simulink model "Simulink_Tutorial_Youtube"  (R2022b)
settings: Solver=FixedStepAuto  StartTime=0.0  StopTime=10  FixedStep=1  RelTol=1e-3
model workspace (MAT data in the model file):
  Sig = Simulink.Signal
  Sig.DataType = 'auto'
  Sig.Dimensions = -1
  Sig.DimensionsMode = 'auto'
  Sig.Complexity = 'auto'
  Sig.SampleTime = -1
  Sig.SamplingMode = 'auto'
  pi = Simulink.Parameter
  pi.Value = 3.14
  pi.DataType = 'double'
  pi.Complexity = 'real'
  pi.Dimensions = [1 1]
undefined symbols (not defined in the file or in its folder): sigbuilder_block, valueOfCounter
libraries: simulink x15, simulink_extras x1, lib_sample x1, dspsigops x1, SignalEditorBlockLib x1
settings Model: Creator=mohsa  LastModifiedBy=mohsa

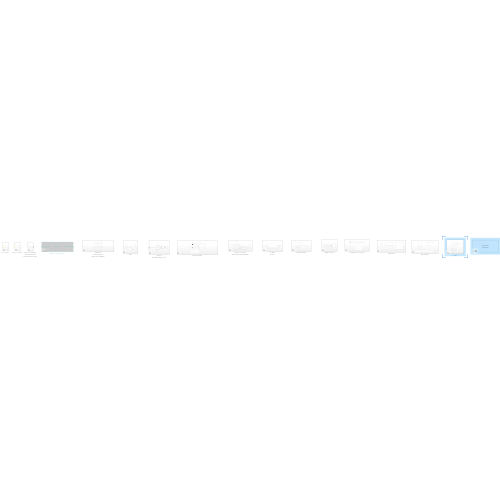
[thumbnail: Simulink's stored preview of the top-level diagram]
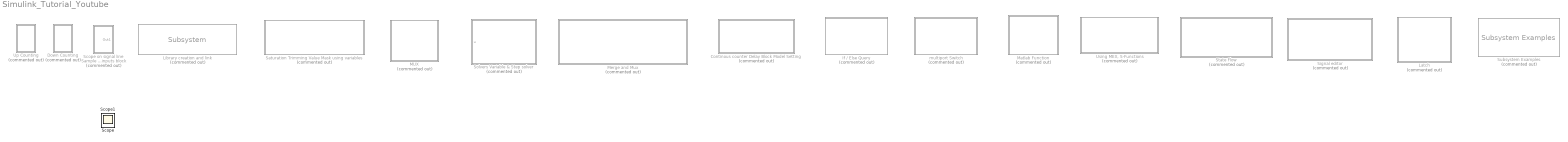
== system Simulink_Tutorial_Youtube ==
  Continous counter Delay Block Model Setting : Subsystem  Commented=on
  Down Counting : Subsystem  Commented=on
  "If / Else Query " : Subsystem  Commented=on
  Latch : Subsystem  Commented=on
  Library creation and link : lib_sample/Subsystem  Commented=on
      settings: LibrarySourceBlock=lib_sample2/Subsystem
  MUX : Subsystem  Commented=on
  Matlab Function : Subsystem  Commented=on
  Merge and Mux : Subsystem  Commented=on
  Saturation Trimming Value Mask using variables : Subsystem  Commented=on
  Scope on signal line Sample and hold Discreate inputs block : Subsystem  Commented=on
  Signal editor : Subsystem  Commented=on
  "Solvers Variable & Step solver " : Subsystem  Commented=on
  State Flow : Subsystem  Commented=on
  Subsystem Examples : simulink/Ports & Subsystems/Subsystem Examples  Commented=on
  Up Counting : Subsystem  Commented=on
  "Using MEX, S-Functions " : Subsystem  Commented=on
  multiport Switch : Subsystem  Commented=on
  Scope : Scope
  Scope1 : Scope

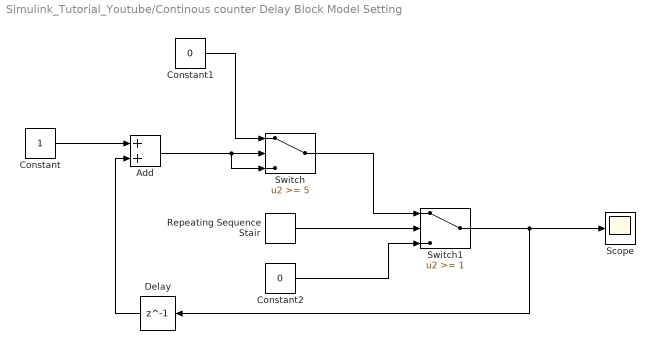
== system Simulink_Tutorial_Youtube/Continous counter Delay Block Model Setting ==
  Add : Sum
  Constant : Constant
  Constant1 : Constant  Value=0
  Constant2 : Constant  Value=0
  Delay : Delay  DelayLength=1
  Repeating Sequence Stair : simulink/Sources/Repeating Sequence Stair  OutValues=[1 ].'  tsamp=-1  OutMin=[]  OutMax=[]  OutDataTypeStr=double  OutputDataTypeScalingMode=double  OutDataType=fixdt(0,8)  ConRadixGroup=Best Precision: Vector-wise  OutScaling=2^-12
  Scope : Scope
  Switch : Switch  Threshold=5  SaturateOnIntegerOverflow=off  InputSameDT=off
  Switch1 : Switch  Threshold=1  SaturateOnIntegerOverflow=off  InputSameDT=off
  wires:
  Constant2/1 -> Switch1/3
  Repeating Sequence Stair/1 -> Switch1/2
  Switch/1 -> Switch1/1
  Constant1/1 -> Switch/1
  Add/1 -> Switch/3, Switch/2
  Constant/1 -> Add/1
  Switch1/1 -> Delay/1, Scope/1
  Delay/1 -> Add/2

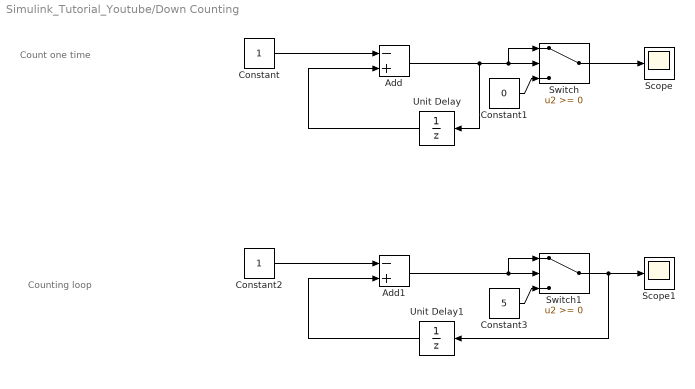
== system Simulink_Tutorial_Youtube/Down Counting ==
  note: Count one time
  note: Counting loop
  Add : Sum  Inputs=-+
  Add1 : Sum  Inputs=-+
  Constant : Constant
  Constant1 : Constant  Value=0
  Constant2 : Constant
  Constant3 : Constant  Value=5
  Scope : Scope
  Scope1 : Scope
  Switch : Switch  SaturateOnIntegerOverflow=off  InputSameDT=off
  Switch1 : Switch  SaturateOnIntegerOverflow=off  InputSameDT=off
  Unit Delay : UnitDelay  InitialCondition=valueOfCounter+1  SampleTime=-1  HasFrameUpgradeWarning=on
  Unit Delay1 : UnitDelay  InitialCondition=valueOfCounter+1  SampleTime=-1  HasFrameUpgradeWarning=on
  wires:
  Unit Delay/1 -> Add/2
  Constant/1 -> Add/1
  Switch/1 -> Scope/1
  Add/1 -> Unit Delay/1, Switch/1, Switch/2
  Constant1/1 -> Switch/3
  Constant3/1 -> Switch1/3
  Add1/1 -> Switch1/2, Switch1/1
  Switch1/1 -> Unit Delay1/1, Scope1/1
  Constant2/1 -> Add1/1
  Unit Delay1/1 -> Add1/2

== system Simulink_Tutorial_Youtube/If // Else Query  ==
  Repeating Sequence Stair : simulink/Sources/Repeating Sequence Stair  OutValues=[0:10:360].'  tsamp=-1  OutMin=[]  OutMax=[]  OutDataTypeStr=double  OutputDataTypeScalingMode=double  OutDataType=fixdt(0,8)  ConRadixGroup=Best Precision: Vector-wise  OutScaling=2^-12
  Scope : Scope  NumInputPorts=2
  Subsystem : Subsystem  mask{upperVal=3*pi/2, lowerVal=pi/2}
      mask prompts: upperVal "upper"; lowerVal "lower"
  wires:
  Repeating Sequence Stair/1 -> Scope/2, Subsystem/1(In1)
  Subsystem/1(Out1) -> Scope/1

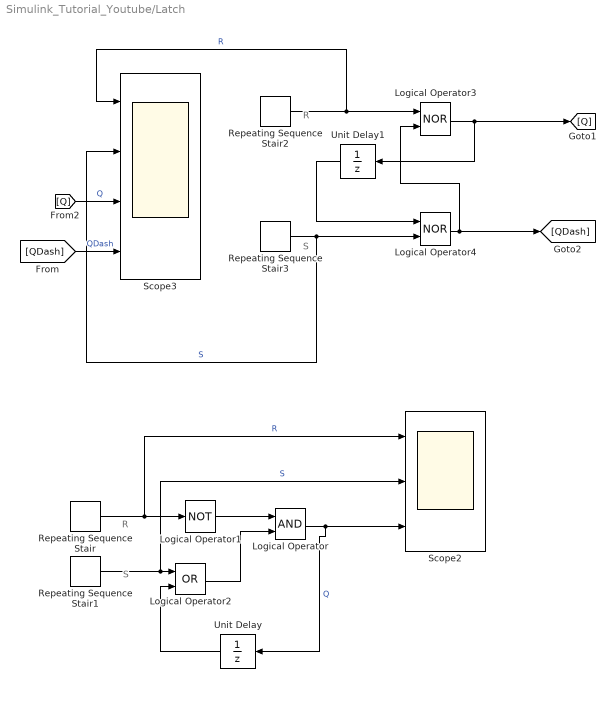
== system Simulink_Tutorial_Youtube/Latch ==
  note: S
  note: R
  note: R
  note: S
  Logical Operator : Logic  AllPortsSameDT=off  OutDataTypeStr=boolean
  Logical Operator1 : Logic  Operator=NOT  AllPortsSameDT=off  OutDataTypeStr=boolean
  Logical Operator2 : Logic  Operator=OR  AllPortsSameDT=off  OutDataTypeStr=boolean
  Logical Operator3 : Logic  Operator=NOR  AllPortsSameDT=off  OutDataTypeStr=boolean
  Logical Operator4 : Logic  Operator=NOR  AllPortsSameDT=off  OutDataTypeStr=boolean
  Repeating Sequence Stair : simulink/Sources/Repeating Sequence Stair  OutValues=[0 1 0 0 0 0 0].'  tsamp=-1  OutMin=[]  OutMax=[]  OutDataTypeStr=double  OutputDataTypeScalingMode=double  OutDataType=fixdt(0,8)  ConRadixGroup=Best Precision: Vector-wise  OutScaling=2^-12
  Repeating Sequence Stair1 : simulink/Sources/Repeating Sequence Stair  OutValues=[0 0 0 0 0 1 0].'  tsamp=-1  OutMin=[]  OutMax=[]  OutDataTypeStr=double  OutputDataTypeScalingMode=double  OutDataType=fixdt(0,8)  ConRadixGroup=Best Precision: Vector-wise  OutScaling=2^-12
  Repeating Sequence Stair2 : simulink/Sources/Repeating Sequence Stair  OutValues=[0 1 0 0 0 0 0].'  tsamp=-1  OutMin=[]  OutMax=[]  OutDataTypeStr=double  OutputDataTypeScalingMode=double  OutDataType=fixdt(0,8)  ConRadixGroup=Best Precision: Vector-wise  OutScaling=2^-12
  Repeating Sequence Stair3 : simulink/Sources/Repeating Sequence Stair  OutValues=[0 0 0 0 0 1 0].'  tsamp=-1  OutMin=[]  OutMax=[]  OutDataTypeStr=double  OutputDataTypeScalingMode=double  OutDataType=fixdt(0,8)  ConRadixGroup=Best Precision: Vector-wise  OutScaling=2^-12
  Scope2 : Scope  NumInputPorts=3
  Scope3 : Scope  NumInputPorts=4
  Unit Delay : UnitDelay  SampleTime=-1  HasFrameUpgradeWarning=on
  Unit Delay1 : UnitDelay  InitialCondition=1  SampleTime=-1  HasFrameUpgradeWarning=on
  wires:
  Logical Operator/1 -> Unit Delay/1, Scope2/3  "Q"
  Repeating Sequence Stair2/1 -> Scope3/1, Logical Operator3/1  "R"
  Repeating Sequence Stair/1 -> Scope2/1, Logical Operator1/1  "R"
  Logical Operator2/1 -> Logical Operator/2
  Unit Delay/1 -> Logical Operator2/2
  Logical Operator4/1 -> Logical Operator3/2, [QDash]
  Repeating Sequence Stair3/1 -> Scope3/2, Logical Operator4/2  "S"
  Repeating Sequence Stair1/1 -> Scope2/2, Logical Operator2/1  "S"
  Logical Operator3/1 -> Unit Delay1/1, [Q]
  [Q] -> Scope3/3  "Q"
  Logical Operator1/1 -> Logical Operator/1
  [QDash] -> Scope3/4  "QDash"
  Unit Delay1/1 -> Logical Operator4/1

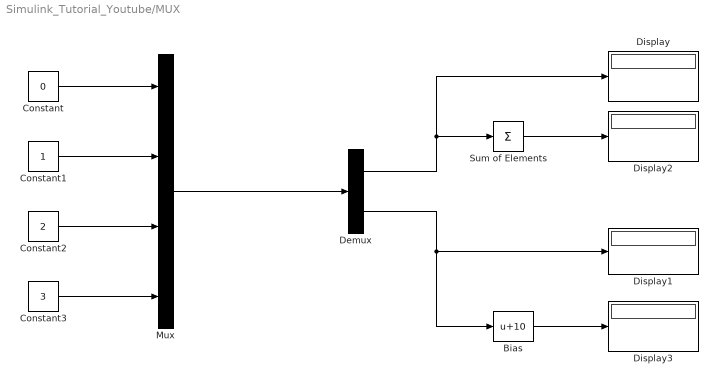
== system Simulink_Tutorial_Youtube/MUX ==
  Bias : Bias  Bias=10  SaturateOnIntegerOverflow=off
  Constant : Constant  Value=0
  Constant1 : Constant
  Constant2 : Constant  Value=2
  Constant3 : Constant  Value=3
  Demux : Demux  Outputs=2
  Display{,1..3} (4 alike) : Display
  Mux : Mux
  Sum of Elements : Sum  Inputs=+
  wires:
  Constant/1 -> Mux/1
  Constant1/1 -> Mux/2
  Constant2/1 -> Mux/3
  Constant3/1 -> Mux/4
  Mux/1 -> Demux/1
  Demux/1 -> Sum of Elements/1, Display/1
  Demux/2 -> Bias/1, Display1/1
  Sum of Elements/1 -> Display2/1
  Bias/1 -> Display3/1

== system Simulink_Tutorial_Youtube/Matlab Function ==
  MATLAB Function : MATLAB Function  TreatAsAtomicUnit=on
  Repeating Sequence Stair : simulink/Sources/Repeating Sequence Stair  OutValues=[0:10:50].'  tsamp=-1  OutMin=[]  OutMax=[]  OutDataTypeStr=double  OutputDataTypeScalingMode=double  OutDataType=fixdt(0,8)  ConRadixGroup=Best Precision: Vector-wise  OutScaling=2^-12
  Scope : Scope  NumInputPorts=4
  wires:
  Repeating Sequence Stair/1 -> Scope/1, MATLAB Function/1(u)
  MATLAB Function/1(x) -> Scope/2
  MATLAB Function/2(y) -> Scope/3
  MATLAB Function/3(z) -> Scope/4

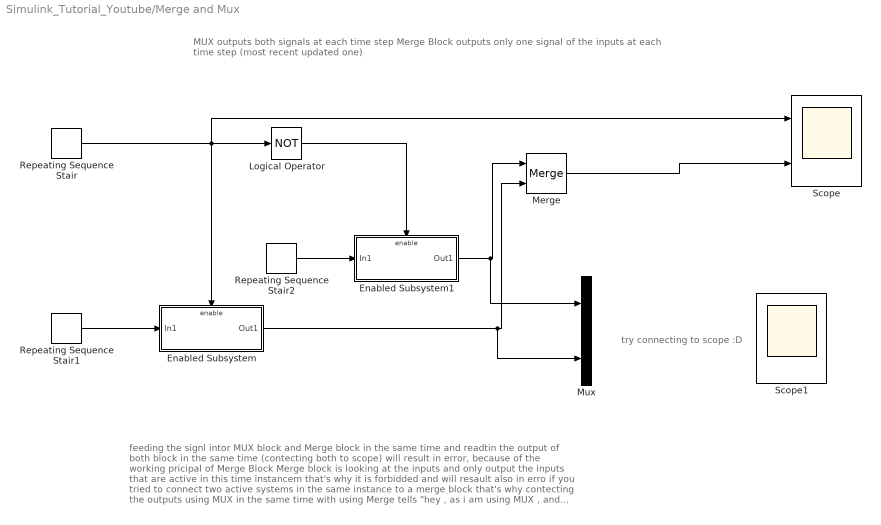
== system Simulink_Tutorial_Youtube/Merge and Mux ==
  note: MUX outputs both signals at each time step
      | Merge Block outputs only one signal of the inputs at each time step (most recent updated one)
  note: try connecting to scope :D
  note: feeding the signl intor MUX block and Merge block in the same time and readtin the output of both block in the same time (contecting both to scope)
      | will result in error, because of the working pricipal of Merge Block
      | Merge block is looking at the inputs and only output the inputs that are active in this time instancem that's why it is forbidded and will resault also in erro if you tried to connect two active systems in the same instance to a merge block
      | that's why contecting the outputs using MUX in the same time with using Merge tells "hey , as i am using MUX , and output it to a scope , then I need to look up the systems singals each time step". the solver will try to do though, in the same time of evaluating which system is working among the Merge Block inputs, it  will figure out that both must be working in the same time step and Merge Block will crash as it only passes one signal which is the signal of the currently working block in each time step (instance).
  Enabled Subsystem : Subsystem  TreatAsAtomicUnit=on
  Enabled Subsystem1 : Subsystem  TreatAsAtomicUnit=on
  Logical Operator : Logic  Operator=NOT  AllPortsSameDT=off  OutDataTypeStr=boolean
  Merge : Merge
  Mux : Mux  Inputs=2
  Repeating Sequence Stair : simulink/Sources/Repeating Sequence Stair  OutValues=[0 0 0].'  tsamp=-1  OutMin=[]  OutMax=[]  OutDataTypeStr=double  OutputDataTypeScalingMode=double  OutDataType=fixdt(0,8)  ConRadixGroup=Best Precision: Vector-wise  OutScaling=2^-12
  Repeating Sequence Stair1 : simulink/Sources/Repeating Sequence Stair  OutValues=[1 0].'  tsamp=-1  OutMin=[]  OutMax=[]  OutDataTypeStr=double  OutputDataTypeScalingMode=double  OutDataType=fixdt(0,8)  ConRadixGroup=Best Precision: Vector-wise  OutScaling=2^-12
  Repeating Sequence Stair2 : simulink/Sources/Repeating Sequence Stair  OutValues=[1 0].'  tsamp=-1  OutMin=[]  OutMax=[]  OutDataTypeStr=double  OutputDataTypeScalingMode=double  OutDataType=fixdt(0,8)  ConRadixGroup=Best Precision: Vector-wise  OutScaling=2^-12
  Scope : Scope  NumInputPorts=2
  Scope1 : Scope
  wires:
  Repeating Sequence Stair1/1 -> Enabled Subsystem/1(In1)
  Repeating Sequence Stair/1 -> Scope/1, Enabled Subsystem/Enable, Logical Operator/1
  Logical Operator/1 -> Enabled Subsystem1/Enable
  Repeating Sequence Stair2/1 -> Enabled Subsystem1/1(In1)
  Enabled Subsystem1/1(Out1) -> Mux/1, Merge/1
  Enabled Subsystem/1(Out1) -> Mux/2, Merge/2
  Merge/1 -> Scope/2

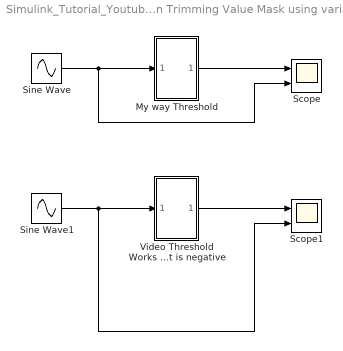
== system Simulink_Tutorial_Youtube/Saturation Trimming Value Mask using variables ==
  My way Threshold : Subsystem  mask(Limits){upper_limit=13, lower_limit=-13}
  Scope : Scope  NumInputPorts=2
  Scope1 : Scope  NumInputPorts=2
  Sine Wave : Sin  Amplitude=15  Frequency=2  SampleTime=0
  Sine Wave1 : Sin  Amplitude=15  Frequency=2  SampleTime=0
  Video Threshold Works only and only if lower limit is negative : Subsystem  mask(Limits){upper_limit=[], lower_limit=-2}
  wires:
  Sine Wave/1 -> Scope/2, My way Threshold/1(In1)
  My way Threshold/1(Out1) -> Scope/1
  Video Threshold Works only and only if lower limit is negative/1(Out1) -> Scope1/1
  Sine Wave1/1 -> Scope1/2, Video Threshold Works only and only if lower limit is negative/1(In1)

== system Simulink_Tutorial_Youtube/Scope on signal line Sample and hold Discreate inputs block ==
  Repeating Sequence Stair : simulink/Sources/Repeating Sequence Stair  OutValues=[1 0].'  tsamp=-1  OutMin=[]  OutMax=[]  OutDataTypeStr=double  OutputDataTypeScalingMode=double  OutDataType=fixdt(0,8)  ConRadixGroup=Best Precision: Vector-wise  OutScaling=2^-12
  Sample and Hold : dspsigops/Sample and Hold  trig=Rising edge  initCond=0  latchinput=off
  Sine Wave : Sin  Amplitude=5  SampleTime=0
  Out1 : Outport
  wires:
  Sample and Hold/1 -> Out1/1
  Sine Wave/1 -> Sample and Hold/1
  Repeating Sequence Stair/1 -> Sample and Hold/Trigger

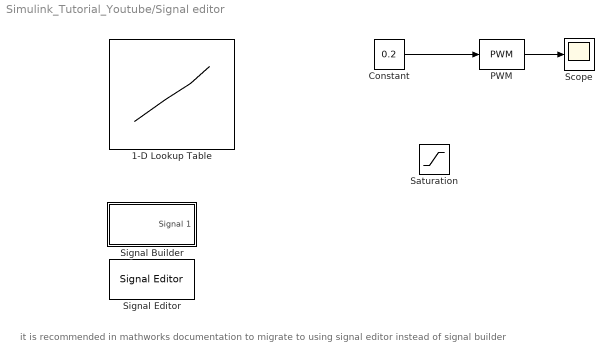
== system Simulink_Tutorial_Youtube/Signal editor ==
  note: it is recommended in mathworks documentation to migrate to using signal editor instead of signal builder
  1-D Lookup Table : Lookup_n-D  NumberOfTableDimensions=1  BreakpointsForDimension1=[0.5:0.04:4.5]  Table=[0:1:100]  InternalRulePriority=Speed  RndMeth=Simplest
  Constant : Constant  Value=0.2
  PWM : simulink/Discontinuities/PWM  DisableCoverage=on  Period=1  InitialDelay=0  DisallowZeroDutyCycle=off  RunAtFixedTimeIntervals=on  SampleTime=0.1
  Saturation : Saturate
  Scope : Scope
  Signal Builder : Subsystem  Tag=STV Subsys  LoadFcn=sigbuilder_block('load');  StartFcn=sigbuilder_block('start');  StopFcn=sigbuilder_block('stop');  ClipboardFcn=sigbuilder_block('clipboard');  mask(Sigbuilder block){tuvar=[0:10]}
      mask help: Simulink:masks:SigbuilderBlock_MD
      mask init:
      | if ~strcmp(get_param(bdroot(gcbh),'SimulationStatus'),'stopped') tuvar = sigbuilder_block('maskInit'); end
      settings: CopyFcn=sigbuilder_block('copy');  DeleteFcn=sigbuilder_block('delete');  ModelCloseFcn=sigbuilder_block('modelClose');  PreSaveFcn=sigbuilder_block('preSave');  PauseFcn=sigbuilder_block('pause');  ContinueFcn=sigbuilder_block('continue');  NameChangeFcn=sigbuilder_block('namechange');  OpenFcn=sigbuilder_block('open',[437.6 199.2 550.4 400 ]);  CloseFcn=sigbuilder_block('close');
      mask Display: plot(0, 0, 100, 100,[2, 2, 32, 32, 2], [68, 8, 8, 68, 68],[32, 2], [38, 38], [32, 19, 2],[53, 60, 44], [32, 17, 17, 2],[16, 16, 31, 31]);txt = getActiveGroup(gcbh);text(2, 100, txt,'verticalAlignment', 'top');
  Signal Editor : SignalEditorBlockLib/Signal Editor  FileName=untitled.mat  ActiveScenario=Scenario  ActiveSignal=Signal 1  IsBus=off  OutputBusObjectStr=Bus: BusObject  SampleTime=0  Interpolate=off  ZeroCross=off  OutputAfterFinalValue=Setting to zero  Unit=inherit  PreserveSignalName=on
  wires:
  Constant/1 -> PWM/1
  PWM/1 -> Scope/1

== system Simulink_Tutorial_Youtube/Solvers Variable & Step solver  ==
  u : Inport
  Constant : Constant
  Constant1 : Constant  Value=0
  Scope2 : Scope
  Switch : Switch  SaturateOnIntegerOverflow=off  InputSameDT=off
  wires:
  u/1 -> Switch/2
  Switch/1 -> Scope2/1
  Constant/1 -> Switch/1
  Constant1/1 -> Switch/3

== system Simulink_Tutorial_Youtube/State Flow ==
  Chart : Stateflow chart  TreatAsAtomicUnit=on
  "Some notes " : Subsystem
  this system outputs any value above 5.5 and output zero for value less or  equal 5.5 and outputs -1 for negative inputs : Subsystem

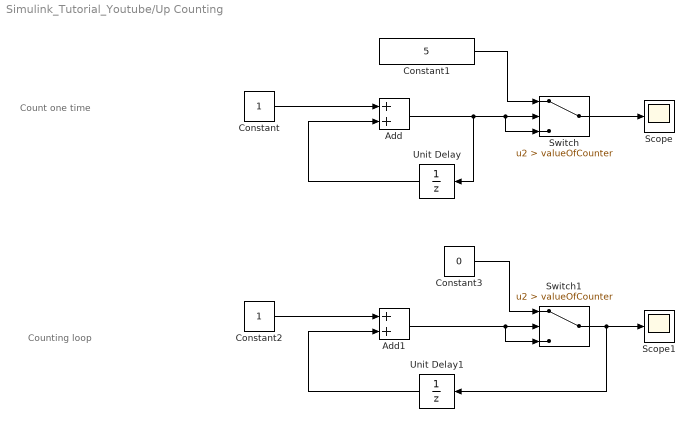
== system Simulink_Tutorial_Youtube/Up Counting ==
  note: Counting loop
  note: Count one time
  Add : Sum
  Add1 : Sum
  Constant : Constant
  Constant1 : Constant  Value=5
  Constant2 : Constant
  Constant3 : Constant  Value=0
  Scope : Scope
  Scope1 : Scope
  Switch : Switch  Criteria=u2 > Threshold  Threshold=valueOfCounter  SaturateOnIntegerOverflow=off  InputSameDT=off
  Switch1 : Switch  Criteria=u2 > Threshold  Threshold=valueOfCounter  SaturateOnIntegerOverflow=off  InputSameDT=off
  Unit Delay : UnitDelay  InitialCondition=-1  SampleTime=-1  HasFrameUpgradeWarning=on
  Unit Delay1 : UnitDelay  InitialCondition=-1  SampleTime=-1  HasFrameUpgradeWarning=on
  wires:
  Add/1 -> Unit Delay/1, Switch/3, Switch/2
  Switch/1 -> Scope/1
  Constant/1 -> Add/1
  Unit Delay/1 -> Add/2
  Constant1/1 -> Switch/1
  Constant3/1 -> Switch1/1
  Unit Delay1/1 -> Add1/2
  Constant2/1 -> Add1/1
  Switch1/1 -> Unit Delay1/1, Scope1/1
  Add1/1 -> Switch1/2, Switch1/3

== system Simulink_Tutorial_Youtube/Using MEX, S-Functions  ==
  note: files related to this:
      |
      | S_Function_trial.m
      | HeaderFileName.h
      | SrcFileName.c
      | my_S_Func.mexw64
      | my_S_Func.c
  Constant : Constant  Value=3.5
  Constant1 : Constant  Value=1.5
  Display : Display
  S-Function : S-Function  FunctionName=my_S_Func  SFunctionDeploymentMode=off  EnableBusSupport=off
  wires:
  Constant1/1 -> S-Function/2
  Constant/1 -> S-Function/1
  S-Function/1 -> Display/1

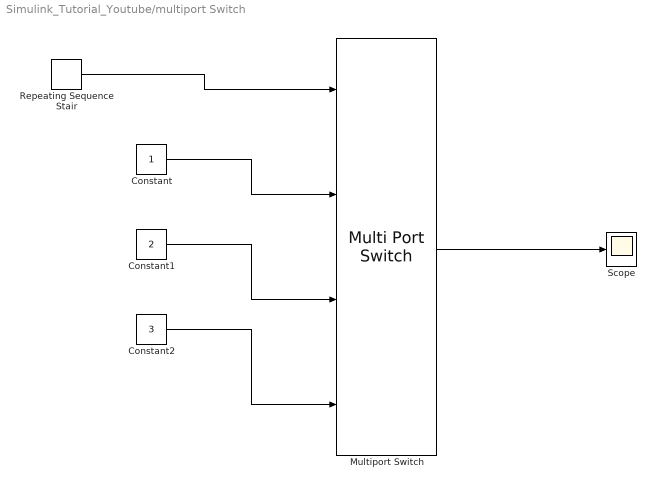
== system Simulink_Tutorial_Youtube/multiport Switch ==
  Constant : Constant
  Constant1 : Constant  Value=2
  Constant2 : Constant  Value=3
  Multiport Switch : MultiPortSwitch  DataPortIndices={1,2,20}  SaturateOnIntegerOverflow=off  InputSameDT=off
  Repeating Sequence Stair : simulink/Sources/Repeating Sequence Stair  OutValues=[1 3 2 1 3 2 3 2 1 1 2 3].'  tsamp=-1  OutMin=[]  OutMax=[]  OutDataTypeStr=double  OutputDataTypeScalingMode=double  OutDataType=fixdt(0,8)  ConRadixGroup=Best Precision: Vector-wise  OutScaling=2^-12
  Scope : Scope
  wires:
  Repeating Sequence Stair/1 -> Multiport Switch/1
  Constant/1 -> Multiport Switch/2
  Constant1/1 -> Multiport Switch/3
  Constant2/1 -> Multiport Switch/4
  Multiport Switch/1 -> Scope/1

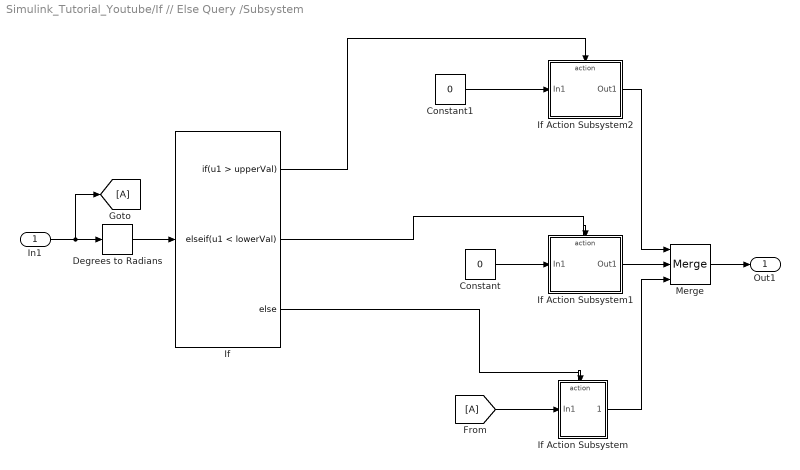
== system Simulink_Tutorial_Youtube/If // Else Query /Subsystem ==
  In1 : Inport
  Constant : Constant  Value=0
  Constant1 : Constant  Value=0
  Degrees to Radians : simulink_extras/Transformations/Degrees to Radians
  From : From
  Goto : Goto
  If : If  IfExpression=u1 > upperVal  ElseIfExpressions=u1 < lowerVal
  If Action Subsystem : Subsystem  TreatAsAtomicUnit=on
  If Action Subsystem1 : Subsystem  TreatAsAtomicUnit=on
  If Action Subsystem2 : Subsystem  TreatAsAtomicUnit=on
  Merge : Merge  Inputs=3
  Out1 : Outport
  wires:
  If/2 -> If Action Subsystem1/Action
  In1/1 -> Degrees to Radians/1, Goto/1
  From/1 -> If Action Subsystem/1(In1)
  Degrees to Radians/1 -> If/1
  Constant1/1 -> If Action Subsystem2/1(In1)
  If/1 -> If Action Subsystem2/Action
  If/3 -> If Action Subsystem/Action
  Constant/1 -> If Action Subsystem1/1(In1)
  If Action Subsystem2/1(Out1) -> Merge/1
  If Action Subsystem1/1(Out1) -> Merge/2
  If Action Subsystem/1(Out1) -> Merge/3
  Merge/1 -> Out1/1

== system Simulink_Tutorial_Youtube/Merge and Mux/Enabled Subsystem ==
  In1 : Inport
  Enable : EnablePort
  Out1 : Outport
  wires:
  In1/1 -> Out1/1

== system Simulink_Tutorial_Youtube/Merge and Mux/Enabled Subsystem1 ==
  In1 : Inport
  Enable : EnablePort
  Out1 : Outport
  wires:
  In1/1 -> Out1/1

== system Simulink_Tutorial_Youtube/Saturation Trimming Value Mask using variables/My way Threshold ==
  In1 : Inport
  Constant : Constant  Value=lower_limit
  Constant1 : Constant  Value=upper_limit
  Switch : Switch  Criteria=u2 > Threshold  Threshold=lower_limit  SaturateOnIntegerOverflow=off  InputSameDT=off
  Switch1 : Switch  Criteria=u2 > Threshold  Threshold=upper_limit  SaturateOnIntegerOverflow=off  InputSameDT=off
  Out1 : Outport
  wires:
  Switch/1 -> Switch1/3, Switch1/2
  In1/1 -> Switch/2, Switch/1
  Constant/1 -> Switch/3
  Switch1/1 -> Out1/1
  Constant1/1 -> Switch1/1

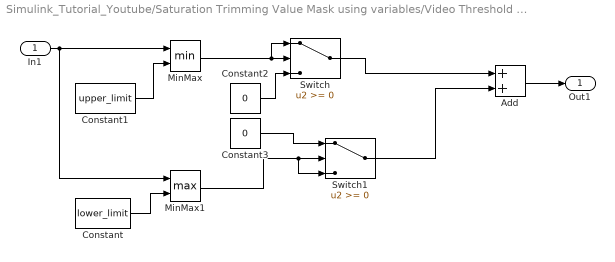
== system Simulink_Tutorial_Youtube/Saturation Trimming Value Mask using variables/Video Threshold Works only and only if lower limit is negative ==
  In1 : Inport
  Add : Sum
  Constant : Constant  Value=lower_limit
  Constant1 : Constant  Value=upper_limit
  Constant2 : Constant  Value=0
  Constant3 : Constant  Value=0
  MinMax : MinMax  Inputs=2
  MinMax1 : MinMax  Function=max  Inputs=2
  Switch : Switch  SaturateOnIntegerOverflow=off  InputSameDT=off
  Switch1 : Switch  SaturateOnIntegerOverflow=off  InputSameDT=off
  Out1 : Outport
  wires:
  In1/1 -> MinMax1/1, MinMax/1
  Constant/1 -> MinMax1/2
  Constant1/1 -> MinMax/2
  Add/1 -> Out1/1
  MinMax/1 -> Switch/1, Switch/2
  Switch/1 -> Add/1
  Constant2/1 -> Switch/3
  Switch1/1 -> Add/2
  Constant3/1 -> Switch1/1
  MinMax1/1 -> Switch1/3, Switch1/2

== system Simulink_Tutorial_Youtube/Signal editor/Signal Builder ==
  Demux : Demux  Tag=STV Demux  Outputs=1
      settings: DisplayOption=none
  FromWs : FromWorkspace  Tag=STV FromWs  VariableName=tuvar
      SigBuilderData=|
      | common.afterFinalStr = 'Extrapolate'
      | common.sampleTime = 0
      | dataSet.timeRange = [0 10]
      | dataSet.name = 'Group 1'
      | sbobj.Groups.Name = 'Group 1'
      | sbobj.Groups.Signals.Name = 'Signal 1'
      | sbobj.Groups.Signals.XData = [0 4 4 6 6 10]
      | sbobj.Groups.Signals.YData = [0 0 1 1 0 0]
  Signal 1 : Outport  Tag=STV Outport
  wires:
  Demux/1 -> Signal 1/1
  FromWs/1 -> Demux/1

== system Simulink_Tutorial_Youtube/State Flow/Some notes  ==
  note: If you have a transition that exits a state based on a condition that evaluates to TRUE , and that transition leads to a junction point where none of the outgoing transitions have a condition that evaluates to TRUE , the behavior depends on the solver settings in your Simulink model.
      | Deterministic Solver:
      | If you are using a deterministic solver, such as a fixed-step solver, the solver will choose one of the outgoing transitions randomly. The choice may vary between simulation runs or between solver steps within a single simulation run.
      | Stochastic Solver:
      | If you are using a stochastic solver, such as a variable-step solver, the solver will handle the situation differently. It may take into account various factors, such as the probabilities associated with the transitions, to make a probabilistic choice. The specific behavior may depend on the configuration of the solver and the settings you have defined.
      | In both cases, the behavior might not be deterministic or predictable, especially in situations where multiple transitions are eligible for execution but none of them have conditions that evaluate to TRUE . It is important to note that this behavior may not be desired and could lead to unexpected results.
      | To avoid such ambiguities and ensure deterministic behavior, it is recommended to define at least one outgoing transition from the junction point with a condition that evaluates to TRUE or use a default transition that captures the remaining cases. This way, you can ensure that the state machine follows a specific path even when none of the conditions of the outgoing transitions are met.
      | Carefully designing the conditions and transitions within your state machine, including the use of default transitions or guard conditions, will help you achieve the desired behavior and avoid ambiguities or unexpected outcomes.
  note: Systems Types:
      | Enabled System : entering system (start executing) requires a specific key (condition, Polling) to enable the system
      | Triggered System : entering system is done depending on specific timing schedual
      | Event System : entering system (start executing) requires a specific key (Event, Interrupt) to enable the system
      |
      | Temporal Logic:
      | system that exist in a state for specific period (absolute - relative timing)
      |
      | State machine types:
      | Mealy : Actions in States only, Conditions on transaitions only
      | Moore : Conditions and Actions are in the transaitions only
      | Classic : Conditions are in transations only. Actions could be in both transations and states.
      |
      | Flow Char vs State Flow
      | Flow Chart : starts and ends at specfici points with no memory storage cabailities or any history of event recording. it consist of Junctions and transations only.
      | State Flow : starts and terminates at any point. it has the capability to store memories and record history of events.
      |
      | Functions Types in Stateflow model
      | State-Flow Function : building function using stateflow logic
      | Simulink Function : building functions using simulink blocks inside stateflow chart
      | Matlab Functions : explicitly write matlab or C script inside Stateflow.
      |
      | Execution of Stateflow (Decomposition)
      | there are two types of execution
      | (Parallel | Simulatenously | AND decomposition) : in which multiple different are being executed in the same sample of time
      | (Sequential | Serial | OR decomposition) : in which only one state is active at each time sample and we are transitioning between them using transitions
      |
      | Ex
  note: State flow terms:
      | State : where the current executing stay
      | Entry : is the action being takeing on entering a state (done once)
      | During : is the action that is being doing while in the state itself (done in a loop repeatedly until we leave the state)
      | Exit : is the action that is done on leaving a state (done once)
      |
      | Bind : it is a feature that mostly refer to the data or events being broadcasted from parent states to children states.
      | is also maybe considered as feature in stateflow that establish relationship between stateflow objects (states, variables, ...etc). like and action on the entery point of state (Binding Actions), or transation from one state to another based on specific condition (Binding Conditions).
      |
      | Non Graphical Objects of stateflow:
      | Data Objects : state flow have its own workspace that have internal data objects, however it could utilize external objects from the outer simulink model but it must be defined.
      | ou must define any internal or external data that you use in a Stateflow chart.
      | Event Objects : it is stateflow object that can trigger the whole chart or trigger specific actions in the chart. you can define events that are seen by every object in the scope of the object sending the event, or you may send the event to specific target.
      | Message Objects : they are queued objects that carry data. messages could be sent from one FlowChart to another FLowChart to communicate with each others. it also could be utilized locally by local objects of flowcahrt. messae could be tracked using Sequence Viewer Block.
      |
      | Graphical Objects of stateflow:
      | Junction : point in which charts decide where to go next based on specific conditions. passing junction and reaching some state takes only on sample time .
      |
      | States :
      | the current execution state of the system, we may have one state active (OR decomposition), We may have multiple states active which is (AND decomposition) .
      |
      | Transition:
      |
      | Used to move from one junction to another, or from one state to another or from junction to state and vice versa
      | Trasistion Types :
      | 1- Unconditional transitions ( default transition ) : which is always TRUE and considered the last choice for the solver if all other transitions are False
      | 2- History transition : is type of transition that leads to the state or junction that was previously active.
      | 3- Self Transition : self-transition remains within the same state. It is useful when you want to trigger actions or update variables within a state without exiting and re-entering the state
      | 4- Timeout Transition: A timeout transition is taken after a specified time delay. It allows you to define a time-based transition independent of specific events or conditions.
      | Trasistion Attributes :
      | 1- Execution order : Number presente on the head of the arrow if the state have multiple transitions in the same direction (directions are Out From The State or In To The State)
      | 2- Condition : in [ ] brackets
      | 3- Action : in cuerly { } brackets
      | 4- Event /Message : the Thunder symbole on the transition arrow
      | https://www.youtube.com/watch?v=jr2mKaRR_f4 - https://www.youtube.com/watch?v=qpfXm4FYgVc
  Decomposition AND : Stateflow chart  TreatAsAtomicUnit=on

== system Simulink_Tutorial_Youtube/State Flow/this system outputs any value above 5.5 and output zero for value less or  equal 5.5 and outputs -1 for negative inputs ==
  Chart : Stateflow chart  TreatAsAtomicUnit=on
  Constant : Constant  Value=5.5
  Repeating Sequence Stair : simulink/Sources/Repeating Sequence Stair  OutValues=[1 2 5 6 8 2 9 3 7 8 2 1 -5 4 -3 9 2 -4 5 9].'  tsamp=-1  OutMin=[]  OutMax=[]  OutDataTypeStr=double  OutputDataTypeScalingMode=double  OutDataType=fixdt(0,8)  ConRadixGroup=Best Precision: Vector-wise  OutScaling=2^-12
  Scope : Scope  NumInputPorts=2
  wires:
  Constant/1 -> Chart/2(threshold)
  Repeating Sequence Stair/1 -> Scope/1, Chart/1(inputData)
  Chart/1(outputData) -> Scope/2

== system Simulink_Tutorial_Youtube/If // Else Query /Subsystem/If Action Subsystem ==
  In1 : Inport
  Action Port : ActionPort  ActionPortLabel=else
  Out1 : Outport
  wires:
  In1/1 -> Out1/1

== system Simulink_Tutorial_Youtube/If // Else Query /Subsystem/If Action Subsystem1 ==
  In1 : Inport
  Action Port : ActionPort  ActionPortLabel=elseif(u1 < lowerVal)
  Out1 : Outport
  wires:
  In1/1 -> Out1/1

== system Simulink_Tutorial_Youtube/If // Else Query /Subsystem/If Action Subsystem2 ==
  In1 : Inport
  Action Port : ActionPort  ActionPortLabel=if(u1 > upperVal)
  Out1 : Outport
  wires:
  In1/1 -> Out1/1

== stateflow chart Simulink_Tutorial_Youtube/State Flow/Chart ==
  state A
    en:
    a = a + 1;
  state B
    en:
  (default) -> A
  (junction 11) -> A [order 2]
  A -> (junction 11) : [a==1]{b = b+1;}  /{ c = c + 1;}
  (junction 11) -> B [order 1] : [a==100]{b = b+1;}  /{ c = c + 1;}
  data: a local =0; b local =0; c local =0

== matlab function Simulink_Tutorial_Youtube/Matlab Function/MATLAB Function ==
  data: x output; u input; y output; a input; b input; z output
function [x,y,z] = fcn(u,a,b)

if (u > 30)
    y= 1;
elseif (u < 25 && u > 10)
    y = 2;
else
    y = 3;
end

a= 20;
b = 30;
x = a;
z = b;

== stateflow chart Simulink_Tutorial_Youtube/State Flow/this system outputs any value above 5.5 and output zero for value less or  equal 5.5 and outputs -1 for negative inputs/Chart ==
  (default) -> (junction 1)
  (junction 1) -> (junction 3) [order 1] : [inputData > threshold]
  (junction 1) -> (junction 5) [order 2]
  (junction 3) -> (junction 11) : {outputData = inputData;}
  (junction 5) -> (junction 13) [order 1] : [inputData <= threshold && inputData > 0]
  (junction 5) -> (junction 23) [order 2] : {outputData = -1;}
  (junction 13) -> (junction 20) : {outputData = 0;}
  (junction 20) -> (junction 23)
  (junction 11) -> (junction 20)
  data: inputData input; outputData output; threshold input

== stateflow chart Simulink_Tutorial_Youtube/State Flow/Some notes /Decomposition AND ==
  state State1 [parallel]
    settings: executionOrder=1
    state a
      entry:
      x = 1;
    state b
      entry:
      x = 0;
    (default) -> State1.a
    State1.b -> State1.a : [x == 0]
    State1.a -> State1.b : [x == 1]
  state State2 [parallel]
    settings: executionOrder=2
    state a
      entry:
      x = 1;
    state b
      entry:
      x = 0;
    (default) -> State2.a
    State2.b -> State2.a : [x == 0]
    State2.a -> State2.b : [x == 1]
  data: x local =1
